simulink model "LUT_liver_pancreas_35"  (R2023b)
settings: Solver=FixedStepAuto  StartTime=0  StopTime=10.1  FixedStep=Timegap  RelTol=1e-3
model workspace (MAT data in the model file):
  T1_input = 1.34
(part 3 of 3)

== system LUT_liver_pancreas_35/If Action Subsystem6/If Action Subsystem2/If Action Subsystem9/If Action Subsystem1 ==
  In1 : Inport
  Action Port : ActionPort  ActionPortLabel=elseif( u1 >= 1.915)
  LUT 1.92RR : Lookup_n-D  NumberOfTableDimensions=1  BreakpointsForDimension1=[404.7876;540.8206;633.9575;726.1135;817.552;908.4902;999.0755;1089.407;1179.553;1269.559;1359.459;1449.276;1539.029;1628.729;1718.387;1808.011;1897.606]  Table=[400;500;600;700;800;900;1000;1100;1200;1300;1400;1500;1600;1700;1800;1900;2000]  InternalRulePriority=Speed  RndMeth=Simplest
  Out1 : Outport
  wires:
  In1/1 -> LUT 1.92RR/1
  LUT 1.92RR/1 -> Out1/1

== system LUT_liver_pancreas_35/If Action Subsystem6/If Action Subsystem2/If Action Subsystem9/If Action Subsystem10 ==
  In1 : Inport
  Action Port : ActionPort  ActionPortLabel=if(u1 >= 1.995)
  LUT 2.00RR : Lookup_n-D  NumberOfTableDimensions=1  BreakpointsForDimension1=[404.3841;540.3186;633.3836;725.4083;816.6655;907.3828;997.7171;1087.775;1177.629;1267.33;1356.913;1446.406;1535.826;1625.189;1714.506;1803.784;1893.031]  Table=[400;500;600;700;800;900;1000;1100;1200;1300;1400;1500;1600;1700;1800;1900;2000]  InternalRulePriority=Speed  RndMeth=Simplest
  Out1 : Outport
  wires:
  In1/1 -> LUT 2.00RR/1
  LUT 2.00RR/1 -> Out1/1

== system LUT_liver_pancreas_35/If Action Subsystem6/If Action Subsystem2/If Action Subsystem9/If Action Subsystem11 ==
  In1 : Inport
  Action Port : ActionPort  ActionPortLabel=elseif( u1 >= 1.905)
  LUT 1.91RR : Lookup_n-D  NumberOfTableDimensions=1  BreakpointsForDimension1=[404.8402;540.8879;634.0358;726.2106;817.6743;908.6425;999.2618;1089.63;1179.815;1269.862;1359.804;1449.664;1539.46;1629.205;1718.908;1808.578;1898.219]  Table=[400;500;600;700;800;900;1000;1100;1200;1300;1400;1500;1600;1700;1800;1900;2000]  InternalRulePriority=Speed  RndMeth=Simplest
  Out1 : Outport
  wires:
  In1/1 -> LUT 1.91RR/1
  LUT 1.91RR/1 -> Out1/1

== system LUT_liver_pancreas_35/If Action Subsystem6/If Action Subsystem2/If Action Subsystem9/If Action Subsystem2 ==
  In1 : Inport
  Action Port : ActionPort  ActionPortLabel=else
  LUT 1.90RR : Lookup_n-D  NumberOfTableDimensions=1  BreakpointsForDimension1=[404.8934;540.9562;634.1157;726.3098;817.7992;908.7982;999.4519;1089.858;1180.082;1270.17;1360.155;1450.058;1539.899;1629.689;1719.438;1809.154;1898.841]  Table=[400;500;600;700;800;900;1000;1100;1200;1300;1400;1500;1600;1700;1800;1900;2000]  InternalRulePriority=Speed  RndMeth=Simplest
  Out1 : Outport
  wires:
  In1/1 -> LUT 1.90RR/1
  LUT 1.90RR/1 -> Out1/1

== system LUT_liver_pancreas_35/If Action Subsystem6/If Action Subsystem2/If Action Subsystem9/If Action Subsystem3 ==
  In1 : Inport
  Action Port : ActionPort  ActionPortLabel=elseif( u1 >= 1.925)
  LUT 1.93RR : Lookup_n-D  NumberOfTableDimensions=1  BreakpointsForDimension1=[404.7354;540.7544;633.8807;726.0185;817.4325;908.341;998.8931;1089.189;1179.296;1269.262;1359.121;1448.895;1538.604;1628.261;1717.874;1807.453;1897.003]  Table=[400;500;600;700;800;900;1000;1100;1200;1300;1400;1500;1600;1700;1800;1900;2000]  InternalRulePriority=Speed  RndMeth=Simplest
  Out1 : Outport
  wires:
  In1/1 -> LUT 1.93RR/1
  LUT 1.93RR/1 -> Out1/1

== system LUT_liver_pancreas_35/If Action Subsystem6/If Action Subsystem2/If Action Subsystem9/If Action Subsystem4 ==
  In1 : Inport
  Action Port : ActionPort  ActionPortLabel=elseif( u1 >= 1.935)
  LUT 1.94RR : Lookup_n-D  NumberOfTableDimensions=1  BreakpointsForDimension1=[404.6838;540.6892;633.8054;725.9255;817.3155;908.1951;998.7144;1088.974;1179.044;1268.97;1358.788;1448.521;1538.187;1627.8;1717.37;1806.904;1896.409]  Table=[400;500;600;700;800;900;1000;1100;1200;1300;1400;1500;1600;1700;1800;1900;2000]  InternalRulePriority=Speed  RndMeth=Simplest
  Out1 : Outport
  wires:
  In1/1 -> LUT 1.94RR/1
  LUT 1.94RR/1 -> Out1/1

== system LUT_liver_pancreas_35/If Action Subsystem6/If Action Subsystem2/If Action Subsystem9/If Action Subsystem5 ==
  In1 : Inport
  Action Port : ActionPort  ActionPortLabel=elseif( u1 >= 1.955)
  LUT 1.96RR : Lookup_n-D  NumberOfTableDimensions=1  BreakpointsForDimension1=[404.582;540.5618;633.6592;725.7455;817.0891;907.9124;998.3679;1088.558;1178.554;1268.403;1358.141;1447.791;1537.374;1626.901;1716.384;1805.831;1895.248]  Table=[400;500;600;700;800;900;1000;1100;1200;1300;1400;1500;1600;1700;1800;1900;2000]  InternalRulePriority=Speed  RndMeth=Simplest
  Out1 : Outport
  wires:
  In1/1 -> LUT 1.96RR/1
  LUT 1.96RR/1 -> Out1/1

== system LUT_liver_pancreas_35/If Action Subsystem6/If Action Subsystem2/If Action Subsystem9/If Action Subsystem6 ==
  In1 : Inport
  Action Port : ActionPort  ActionPortLabel=elseif( u1 >= 1.945)
  LUT 1.95RR : Lookup_n-D  NumberOfTableDimensions=1  BreakpointsForDimension1=[404.6326;540.625;633.7316;725.8345;817.201;908.0522;998.5393;1088.764;1178.796;1268.684;1358.461;1448.153;1537.777;1627.347;1716.873;1806.363;1895.824]  Table=[400;500;600;700;800;900;1000;1100;1200;1300;1400;1500;1600;1700;1800;1900;2000]  InternalRulePriority=Speed  RndMeth=Simplest
  Out1 : Outport
  wires:
  In1/1 -> LUT 1.95RR/1
  LUT 1.95RR/1 -> Out1/1

== system LUT_liver_pancreas_35/If Action Subsystem6/If Action Subsystem2/If Action Subsystem9/If Action Subsystem7 ==
  In1 : Inport
  Action Port : ActionPort  ActionPortLabel=elseif( u1 >= 1.965)
  LUT 1.97RR : Lookup_n-D  NumberOfTableDimensions=1  BreakpointsForDimension1=[404.5318;540.4996;633.5882;725.6584;816.9796;907.7756;998.2001;1088.357;1178.316;1268.127;1357.825;1447.436;1536.977;1626.463;1715.903;1805.307;1894.681]  Table=[400;500;600;700;800;900;1000;1100;1200;1300;1400;1500;1600;1700;1800;1900;2000]  InternalRulePriority=Speed  RndMeth=Simplest
  Out1 : Outport
  wires:
  In1/1 -> LUT 1.97RR/1
  LUT 1.97RR/1 -> Out1/1

== system LUT_liver_pancreas_35/If Action Subsystem6/If Action Subsystem2/If Action Subsystem9/If Action Subsystem8 ==
  In1 : Inport
  Action Port : ActionPort  ActionPortLabel=elseif( u1 >= 1.975)
  LUT 1.98RR : Lookup_n-D  NumberOfTableDimensions=1  BreakpointsForDimension1=[404.4821;540.4383;633.5187;725.5732;816.8726;907.6418;998.0357;1088.159;1178.082;1267.856;1357.516;1447.086;1536.587;1626.031;1715.43;1804.792;1894.123]  Table=[400;500;600;700;800;900;1000;1100;1200;1300;1400;1500;1600;1700;1800;1900;2000]  InternalRulePriority=Speed  RndMeth=Simplest
  Out1 : Outport
  wires:
  In1/1 -> LUT 1.98RR/1
  LUT 1.98RR/1 -> Out1/1

== system LUT_liver_pancreas_35/If Action Subsystem6/If Action Subsystem2/If Action Subsystem9/If Action Subsystem9 ==
  In1 : Inport
  Action Port : ActionPort  ActionPortLabel=elseif(u1 >= 1.985)
  LUT 1.99RR : Lookup_n-D  NumberOfTableDimensions=1  BreakpointsForDimension1=[404.4328;540.378;633.4504;725.4899;816.7679;907.5109;997.8747;1087.965;1177.853;1267.59;1357.212;1446.743;1536.203;1625.607;1714.964;1804.284;1893.573]  Table=[400;500;600;700;800;900;1000;1100;1200;1300;1400;1500;1600;1700;1800;1900;2000]  InternalRulePriority=Speed  RndMeth=Simplest
  Out1 : Outport
  wires:
  In1/1 -> LUT 1.99RR/1
  LUT 1.99RR/1 -> Out1/1

== system LUT_liver_pancreas_35/If Action Subsystem6/If Action Subsystem3/If Action Subsystem5/If Action Subsystem1 ==
  In1 : Inport
  Action Port : ActionPort  ActionPortLabel=elseif( u1 >= 0.615)
  LUT 0.62RR : Lookup_n-D  NumberOfTableDimensions=1  BreakpointsForDimension1=[422.6336;583.5736;694.2332;805.1871;916.263;1027.405;1138.585;1249.783;1360.984;1472.171;1583.31;1694.13;1806.172;1917.097;2028.157;2139.213;2250.242]  Table=[400;500;600;700;800;900;1000;1100;1200;1300;1400;1500;1600;1700;1800;1900;2000]  InternalRulePriority=Speed  RndMeth=Simplest
  Out1 : Outport
  wires:
  In1/1 -> LUT 0.62RR/1
  LUT 0.62RR/1 -> Out1/1

== system LUT_liver_pancreas_35/If Action Subsystem6/If Action Subsystem3/If Action Subsystem5/If Action Subsystem10 ==
  In1 : Inport
  Action Port : ActionPort  ActionPortLabel=elseif( u1 >= 0.605)
  LUT 0.61RR : Lookup_n-D  NumberOfTableDimensions=1  BreakpointsForDimension1=[422.9526;584.7206;695.933;807.4484;919.09;1030.799;1142.546;1254.308;1366.068;1477.806;1589.47;1700.311;1813.447;1924.961;2036.559;2148.143;2259.695]  Table=[400;500;600;700;800;900;1000;1100;1200;1300;1400;1500;1600;1700;1800;1900;2000]  InternalRulePriority=Speed  RndMeth=Simplest
  Out1 : Outport
  wires:
  In1/1 -> LUT 0.61RR/1
  LUT 0.61RR/1 -> Out1/1

== system LUT_liver_pancreas_35/If Action Subsystem6/If Action Subsystem3/If Action Subsystem5/If Action Subsystem2 ==
  In1 : Inport
  Action Port : ActionPort  ActionPortLabel=else
  LUT 0.6RR : Lookup_n-D  NumberOfTableDimensions=1  BreakpointsForDimension1=[423.273;585.8952;697.6778;809.7724;921.9972;1034.291;1146.621;1258.963;1371.298;1483.599;1595.782;1705.399;1820.947;1933.043;2045.189;2157.312;2269.393]  Table=[400;500;600;700;800;900;1000;1100;1200;1300;1400;1500;1600;1700;1800;1900;2000]  InternalRulePriority=Speed  RndMeth=Simplest
  Out1 : Outport
  wires:
  In1/1 -> LUT 0.6RR/1
  LUT 0.6RR/1 -> Out1/1

== system LUT_liver_pancreas_35/If Action Subsystem6/If Action Subsystem3/If Action Subsystem5/If Action Subsystem3 ==
  In1 : Inport
  Action Port : ActionPort  ActionPortLabel=elseif( u1 >= 0.625)
  LUT 0.63RR : Lookup_n-D  NumberOfTableDimensions=1  BreakpointsForDimension1=[422.3166;582.4549;692.5789;802.9886;913.5163;1024.109;1134.74;1245.39;1356.046;1466.695;1577.314;1687.781;1799.151;1909.451;2019.985;2130.523;2241.04]  Table=[400;500;600;700;800;900;1000;1100;1200;1300;1400;1500;1600;1700;1800;1900;2000]  InternalRulePriority=Speed  RndMeth=Simplest
  Out1 : Outport
  wires:
  In1/1 -> LUT 0.63RR/1
  LUT 0.63RR/1 -> Out1/1

== system LUT_liver_pancreas_35/If Action Subsystem6/If Action Subsystem3/If Action Subsystem5/If Action Subsystem4 ==
  In1 : Inport
  Action Port : ActionPort  ActionPortLabel=elseif( u1 >= 0.635)
  LUT 0.64RR : Lookup_n-D  NumberOfTableDimensions=1  BreakpointsForDimension1=[422.0023;581.3647;690.97;800.8527;910.8493;1020.909;1131.007;1241.125;1351.253;1461.377;1571.483;1681.509;1785.582;1902.025;2012.044;2122.075;2232.091]  Table=[400;500;600;700;800;900;1000;1100;1200;1300;1400;1500;1600;1700;1800;1900;2000]  InternalRulePriority=Speed  RndMeth=Simplest
  Out1 : Outport
  wires:
  In1/1 -> LUT 0.64RR/1
  LUT 0.64RR/1 -> Out1/1

== system LUT_liver_pancreas_35/If Action Subsystem6/If Action Subsystem3/If Action Subsystem5/If Action Subsystem5 ==
  In1 : Inport
  Action Port : ActionPort  ActionPortLabel=elseif( u1 >= 0.655)
  LUT 0.66RR : Lookup_n-D  NumberOfTableDimensions=1  BreakpointsForDimension1=[421.3837;579.27;687.8874;796.7656;905.7496;1014.793;1123.873;1232.976;1342.09;1451.208;1560.321;1669.408;1778.206;1887.823;1996.844;2105.898;2214.945]  Table=[400;500;600;700;800;900;1000;1100;1200;1300;1400;1500;1600;1700;1800;1900;2000]  InternalRulePriority=Speed  RndMeth=Simplest
  Out1 : Outport
  wires:
  In1/1 -> LUT 0.66RR/1
  LUT 0.66RR/1 -> Out1/1

== system LUT_liver_pancreas_35/If Action Subsystem6/If Action Subsystem3/If Action Subsystem5/If Action Subsystem6 ==
  In1 : Inport
  Action Port : ActionPort  ActionPortLabel=elseif( u1 >= 0.645)
  LUT 0.65RR : Lookup_n-D  NumberOfTableDimensions=1  BreakpointsForDimension1=[421.6912;580.3031;689.4064;798.7787;908.2609;1017.805;1127.386;1236.988;1346.602;1456.216;1565.819;1675.378;1783.464;1894.816;2004.331;2113.868;2223.393]  Table=[400;500;600;700;800;900;1000;1100;1200;1300;1400;1500;1600;1700;1800;1900;2000]  InternalRulePriority=Speed  RndMeth=Simplest
  Out1 : Outport
  wires:
  In1/1 -> LUT 0.65RR/1
  LUT 0.65RR/1 -> Out1/1

== system LUT_liver_pancreas_35/If Action Subsystem6/If Action Subsystem3/If Action Subsystem5/If Action Subsystem7 ==
  In1 : Inport
  Action Port : ActionPort  ActionPortLabel=elseif( u1 >= 0.665)
  LUT 0.67RR : Lookup_n-D  NumberOfTableDimensions=1  BreakpointsForDimension1=[421.0801;578.2651;686.4124;794.8123;903.3138;1011.873;1120.468;1229.085;1337.715;1446.351;1554.985;1663.605;1772.127;1881.043;1989.578;2098.162;2206.742]  Table=[400;500;600;700;800;900;1000;1100;1200;1300;1400;1500;1600;1700;1800;1900;2000]  InternalRulePriority=Speed  RndMeth=Simplest
  Out1 : Outport
  wires:
  In1/1 -> LUT 0.67RR/1
  LUT 0.67RR/1 -> Out1/1

== system LUT_liver_pancreas_35/If Action Subsystem6/If Action Subsystem3/If Action Subsystem5/If Action Subsystem8 ==
  In1 : Inport
  Action Port : ActionPort  ActionPortLabel=elseif(u1 >= 0.675)
  LUT 0.68RR : Lookup_n-D  NumberOfTableDimensions=1  BreakpointsForDimension1=[420.7806;577.2879;684.9805;792.9173;900.9516;1009.041;1117.166;1225.313;1333.473;1441.641;1549.809;1657.97;1766.09;1874.481;1982.528;2090.655;2198.779]  Table=[400;500;600;700;800;900;1000;1100;1200;1300;1400;1500;1600;1700;1800;1900;2000]  InternalRulePriority=Speed  RndMeth=Simplest
  Out1 : Outport
  wires:
  In1/1 -> LUT 0.68RR/1
  LUT 0.68RR/1 -> Out1/1

== system LUT_liver_pancreas_35/If Action Subsystem6/If Action Subsystem3/If Action Subsystem5/If Action Subsystem9 ==
  In1 : Inport
  Action Port : ActionPort  ActionPortLabel=if(u1 >= 0.685)
  LUT 0.69RR : Lookup_n-D  NumberOfTableDimensions=1  BreakpointsForDimension1=[420.4856;576.3379;683.5906;791.0792;898.661;1006.296;1113.964;1221.655;1329.36;1437.073;1544.789;1652.501;1760.195;1862.439;1975.689;2083.371;2191.052]  Table=[400;500;600;700;800;900;1000;1100;1200;1300;1400;1500;1600;1700;1800;1900;2000]  InternalRulePriority=Speed  RndMeth=Simplest
  Out1 : Outport
  wires:
  In1/1 -> LUT 0.69RR/1
  LUT 0.69RR/1 -> Out1/1

== system LUT_liver_pancreas_35/If Action Subsystem6/If Action Subsystem3/If Action Subsystem6/If Action Subsystem1 ==
  In1 : Inport
  Action Port : ActionPort  ActionPortLabel=elseif( u1 >= 0.515)
  LUT 0.52RR : Lookup_n-D  NumberOfTableDimensions=1  BreakpointsForDimension1=[425.7431;596.0299;712.9409;830.2663;947.7614;1065.323;1182.884;1300.384;1417.721;1534.25;1653.44;1770.224;1887.116;2003.896;2120.516;2236.955;2353.2]  Table=[400;500;600;700;800;900;1000;1100;1200;1300;1400;1500;1600;1700;1800;1900;2000]  InternalRulePriority=Speed  RndMeth=Simplest
  Out1 : Outport
  wires:
  In1/1 -> LUT 0.52RR/1
  LUT 0.52RR/1 -> Out1/1

== system LUT_liver_pancreas_35/If Action Subsystem6/If Action Subsystem3/If Action Subsystem6/If Action Subsystem10 ==
  In1 : Inport
  Action Port : ActionPort  ActionPortLabel=elseif( u1 >= 0.505)
  LUT 0.51RR : Lookup_n-D  NumberOfTableDimensions=1  BreakpointsForDimension1=[426.0152;597.3196;714.917;832.9499;951.1599;1069.435;1187.698;1305.881;1423.854;1540.583;1660.719;1778.215;1895.688;2013.001;2130.113;2247.006;2363.667]  Table=[400;500;600;700;800;900;1000;1100;1200;1300;1400;1500;1600;1700;1800;1900;2000]  InternalRulePriority=Speed  RndMeth=Simplest
  Out1 : Outport
  wires:
  In1/1 -> LUT 0.51RR/1
  LUT 0.51RR/1 -> Out1/1

== system LUT_liver_pancreas_35/If Action Subsystem6/If Action Subsystem3/If Action Subsystem6/If Action Subsystem2 ==
  In1 : Inport
  Action Port : ActionPort  ActionPortLabel=else
  LUT 0.50RR : Lookup_n-D  NumberOfTableDimensions=1  BreakpointsForDimension1=[426.2724;598.586;716.8671;835.6082;954.5351;1073.524;1192.49;1311.353;1429.951;1547.041;1667.958;1786.098;1904.115;2021.919;2139.477;2256.768;2373.782]  Table=[400;500;600;700;800;900;1000;1100;1200;1300;1400;1500;1600;1700;1800;1900;2000]  InternalRulePriority=Speed  RndMeth=Simplest
  Out1 : Outport
  wires:
  In1/1 -> LUT 0.50RR/1
  LUT 0.50RR/1 -> Out1/1

== system LUT_liver_pancreas_35/If Action Subsystem6/If Action Subsystem3/If Action Subsystem6/If Action Subsystem3 ==
  In1 : Inport
  Action Port : ActionPort  ActionPortLabel=elseif( u1 >= 0.525)
  LUT 0.53RR : Lookup_n-D  NumberOfTableDimensions=1  BreakpointsForDimension1=[424.9443;594.7286;710.9561;827.5799;944.3669;1061.222;1178.086;1294.904;1411.598;1527.786;1646.232;1762.207;1878.492;1994.71;2110.804;2226.749;2342.533]  Table=[400;500;600;700;800;900;1000;1100;1200;1300;1400;1500;1600;1700;1800;1900;2000]  InternalRulePriority=Speed  RndMeth=Simplest
  Out1 : Outport
  wires:
  In1/1 -> LUT 0.53RR/1
  LUT 0.53RR/1 -> Out1/1

== system LUT_liver_pancreas_35/If Action Subsystem6/If Action Subsystem3/If Action Subsystem6/If Action Subsystem4 ==
  In1 : Inport
  Action Port : ActionPort  ActionPortLabel=elseif( u1 >= 0.535)
  LUT 0.54RR : Lookup_n-D  NumberOfTableDimensions=1  BreakpointsForDimension1=[425.2839;593.4253;708.9767;824.9086;940.9979;1057.157;1173.331;1289.473;1405.522;1521.245;1639.267;1754.228;1869.886;1985.525;2101.069;2216.493;2331.782]  Table=[400;500;600;700;800;900;1000;1100;1200;1300;1400;1500;1600;1700;1800;1900;2000]  InternalRulePriority=Speed  RndMeth=Simplest
  Out1 : Outport
  wires:
  In1/1 -> LUT 0.54RR/1
  LUT 0.54RR/1 -> Out1/1

== system LUT_liver_pancreas_35/If Action Subsystem6/If Action Subsystem3/If Action Subsystem6/If Action Subsystem5 ==
  In1 : Inport
  Action Port : ActionPort  ActionPortLabel=elseif( u1 >= 0.555)
  LUT 0.56RR : Lookup_n-D  NumberOfTableDimensions=1  BreakpointsForDimension1=[424.5481;590.8416;705.0753;819.6628;934.3976;1049.203;1164.034;1278.855;1393.626;1508.247;1621.489;1738.584;1852.937;1967.393;2081.803;2196.135;2310.376]  Table=[400;500;600;700;800;900;1000;1100;1200;1300;1400;1500;1600;1700;1800;1900;2000]  InternalRulePriority=Speed  RndMeth=Simplest
  Out1 : Outport
  wires:
  In1/1 -> LUT 0.56RR/1
  LUT 0.56RR/1 -> Out1/1

== system LUT_liver_pancreas_35/If Action Subsystem6/If Action Subsystem3/If Action Subsystem6/If Action Subsystem6 ==
  In1 : Inport
  Action Port : ActionPort  ActionPortLabel=elseif( u1 >= 0.545)
  LUT 0.55RR : Lookup_n-D  NumberOfTableDimensions=1  BreakpointsForDimension1=[424.8587;592.1276;707.0136;822.2661;937.6706;1053.146;1168.641;1284.117;1399.524;1514.713;1627.08;1746.339;1861.354;1976.403;2091.384;2206.268;2321.04]  Table=[400;500;600;700;800;900;1000;1100;1200;1300;1400;1500;1600;1700;1800;1900;2000]  InternalRulePriority=Speed  RndMeth=Simplest
  Out1 : Outport
  wires:
  In1/1 -> LUT 0.55RR/1
  LUT 0.55RR/1 -> Out1/1

== system LUT_liver_pancreas_35/If Action Subsystem6/If Action Subsystem3/If Action Subsystem6/If Action Subsystem7 ==
  In1 : Inport
  Action Port : ActionPort  ActionPortLabel=elseif( u1 >= 0.565)
  LUT 0.57RR : Lookup_n-D  NumberOfTableDimensions=1  BreakpointsForDimension1=[424.2327;589.5721;703.1683;817.1068;931.1881;1045.34;1159.521;1273.7;1387.844;1501.884;1615.274;1731.006;1844.668;1958.528;2072.366;2186.143;2299.845]  Table=[400;500;600;700;800;900;1000;1100;1200;1300;1400;1500;1600;1700;1800;1900;2000]  InternalRulePriority=Speed  RndMeth=Simplest
  Out1 : Outport
  wires:
  In1/1 -> LUT 0.57RR/1
  LUT 0.57RR/1 -> Out1/1

== system LUT_liver_pancreas_35/If Action Subsystem6/If Action Subsystem3/If Action Subsystem6/If Action Subsystem8 ==
  In1 : Inport
  Action Port : ActionPort  ActionPortLabel=elseif(u1 >= 0.575)
  LUT 0.58RR : Lookup_n-D  NumberOfTableDimensions=1  BreakpointsForDimension1=[423.9142;588.3227;701.2975;814.6039;928.0487;1041.564;1155.111;1268.662;1382.19;1495.645;1608.761;1723.669;1836.569;1949.837;2063.105;2176.326;2289.486]  Table=[400;500;600;700;800;900;1000;1100;1200;1300;1400;1500;1600;1700;1800;1900;2000]  InternalRulePriority=Speed  RndMeth=Simplest
  Out1 : Outport
  wires:
  In1/1 -> LUT 0.58RR/1
  LUT 0.58RR/1 -> Out1/1

== system LUT_liver_pancreas_35/If Action Subsystem6/If Action Subsystem3/If Action Subsystem6/If Action Subsystem9 ==
  In1 : Inport
  Action Port : ActionPort  ActionPortLabel=if(u1 >= 0.585)
  LUT 0.59RR : Lookup_n-D  NumberOfTableDimensions=1  BreakpointsForDimension1=[423.5939;587.0964;699.4665;812.1582;924.9841;1037.88;1150.81;1263.749;1376.673;1489.547;1602.227;1709.092;1828.658;1941.338;2054.041;2166.71;2279.328]  Table=[400;500;600;700;800;900;1000;1100;1200;1300;1400;1500;1600;1700;1800;1900;2000]  InternalRulePriority=Speed  RndMeth=Simplest
  Out1 : Outport
  wires:
  In1/1 -> LUT 0.59RR/1
  LUT 0.59RR/1 -> Out1/1

== system LUT_liver_pancreas_35/If Action Subsystem6/If Action Subsystem3/If Action Subsystem7/If Action Subsystem1 ==
  In1 : Inport
  Action Port : ActionPort  ActionPortLabel=elseif( u1 >= 0.715)
  LUT 0.72RR : Lookup_n-D  NumberOfTableDimensions=1  BreakpointsForDimension1=[419.6278;573.6455;679.6626;785.8906;892.1983;998.5516;1104.935;1211.338;1317.756;1424.183;1530.616;1637.051;1743.486;1849.909;1956.375;2062.793;2169.214]  Table=[400;500;600;700;800;900;1000;1100;1200;1300;1400;1500;1600;1700;1800;1900;2000]  InternalRulePriority=Speed  RndMeth=Simplest
  Out1 : Outport
  wires:
  In1/1 -> LUT 0.72RR/1
  LUT 0.72RR/1 -> Out1/1

== system LUT_liver_pancreas_35/If Action Subsystem6/If Action Subsystem3/If Action Subsystem7/If Action Subsystem10 ==
  In1 : Inport
  Action Port : ActionPort  ActionPortLabel=elseif( u1 >= 0.705)
  LUT 0.71RR : Lookup_n-D  NumberOfTableDimensions=1  BreakpointsForDimension1=[419.909;574.5174;680.9328;787.5675;894.2865;1001.054;1107.852;1214.672;1321.506;1428.349;1535.197;1642.046;1748.892;1855.694;1962.619;2069.446;2176.275]  Table=[400;500;600;700;800;900;1000;1100;1200;1300;1400;1500;1600;1700;1800;1900;2000]  InternalRulePriority=Speed  RndMeth=Simplest
  Out1 : Outport
  wires:
  In1/1 -> LUT 0.71RR/1
  LUT 0.71RR/1 -> Out1/1

== system LUT_liver_pancreas_35/If Action Subsystem6/If Action Subsystem3/If Action Subsystem7/If Action Subsystem2 ==
  In1 : Inport
  Action Port : ActionPort  ActionPortLabel=else
  LUT 0.70RR : Lookup_n-D  NumberOfTableDimensions=1  BreakpointsForDimension1=[420.195;575.4146;682.2417;789.2965;896.4401;1003.634;1110.861;1218.109;1325.372;1432.644;1539.919;1647.194;1754.461;1861.375;1969.055;2076.303;2183.552]  Table=[400;500;600;700;800;900;1000;1100;1200;1300;1400;1500;1600;1700;1800;1900;2000]  InternalRulePriority=Speed  RndMeth=Simplest
  Out1 : Outport
  wires:
  In1/1 -> LUT 0.70RR/1
  LUT 0.70RR/1 -> Out1/1

== system LUT_liver_pancreas_35/If Action Subsystem6/If Action Subsystem3/If Action Subsystem7/If Action Subsystem3 ==
  In1 : Inport
  Action Port : ActionPort  ActionPortLabel=elseif( u1 >= 0.725)
  LUT 0.73RR : Lookup_n-D  NumberOfTableDimensions=1  BreakpointsForDimension1=[419.3512;572.7984;678.4301;784.2641;890.1733;996.1255;1102.106;1208.106;1314.12;1420.143;1526.173;1632.205;1738.239;1844.269;1950.317;2056.338;2162.36]  Table=[400;500;600;700;800;900;1000;1100;1200;1300;1400;1500;1600;1700;1800;1900;2000]  InternalRulePriority=Speed  RndMeth=Simplest
  Out1 : Outport
  wires:
  In1/1 -> LUT 0.73RR/1
  LUT 0.73RR/1 -> Out1/1

== system LUT_liver_pancreas_35/If Action Subsystem6/If Action Subsystem3/If Action Subsystem7/If Action Subsystem4 ==
  In1 : Inport
  Action Port : ActionPort  ActionPortLabel=elseif( u1 >= 0.735)
  LUT 0.74RR : Lookup_n-D  NumberOfTableDimensions=1  BreakpointsForDimension1=[419.0794;571.9752;677.234;782.6864;888.2094;993.7726;1099.362;1204.971;1310.593;1416.224;1521.862;1627.503;1733.147;1838.789;1939.661;2050.073;2155.709]  Table=[400;500;600;700;800;900;1000;1100;1200;1300;1400;1500;1600;1700;1800;1900;2000]  InternalRulePriority=Speed  RndMeth=Simplest
  Out1 : Outport
  wires:
  In1/1 -> LUT 0.74RR/1
  LUT 0.74RR/1 -> Out1/1

== system LUT_liver_pancreas_35/If Action Subsystem6/If Action Subsystem3/If Action Subsystem7/If Action Subsystem5 ==
  In1 : Inport
  Action Port : ActionPort  ActionPortLabel=elseif( u1 >= 0.755)
  LUT 0.76RR : Lookup_n-D  NumberOfTableDimensions=1  BreakpointsForDimension1=[418.5498;570.398;674.9465;779.6711;884.4567;989.2767;1094.12;1198.98;1303.852;1408.734;1513.621;1618.513;1723.407;1828.302;1933.195;2038.092;2142.984]  Table=[400;500;600;700;800;900;1000;1100;1200;1300;1400;1500;1600;1700;1800;1900;2000]  InternalRulePriority=Speed  RndMeth=Simplest
  Out1 : Outport
  wires:
  In1/1 -> LUT 0.76RR/1
  LUT 0.76RR/1 -> Out1/1

== system LUT_liver_pancreas_35/If Action Subsystem6/If Action Subsystem3/If Action Subsystem7/If Action Subsystem6 ==
  In1 : Inport
  Action Port : ActionPort  ActionPortLabel=elseif( u1 >= 0.745)
  LUT 0.75RR : Lookup_n-D  NumberOfTableDimensions=1  BreakpointsForDimension1=[418.8123;571.1753;676.0732;781.156;886.3045;991.4905;1096.701;1201.93;1307.172;1412.423;1517.68;1622.941;1728.204;1833.468;1938.732;2043.993;2149.252]  Table=[400;500;600;700;800;900;1000;1100;1200;1300;1400;1500;1600;1700;1800;1900;2000]  InternalRulePriority=Speed  RndMeth=Simplest
  Out1 : Outport
  wires:
  In1/1 -> LUT 0.75RR/1
  LUT 0.75RR/1 -> Out1/1

== system LUT_liver_pancreas_35/If Action Subsystem6/If Action Subsystem3/If Action Subsystem7/If Action Subsystem7 ==
  In1 : Inport
  Action Port : ActionPort  ActionPortLabel=elseif( u1 >= 0.765)
  LUT 0.77RR : Lookup_n-D  NumberOfTableDimensions=1  BreakpointsForDimension1=[418.2921;569.6426;673.8529;778.2303;882.6638;987.1289;1091.615;1196.117;1300.631;1405.153;1509.682;1614.214;1718.749;1823.285;1927.819;2032.366;2136.897]  Table=[400;500;600;700;800;900;1000;1100;1200;1300;1400;1500;1600;1700;1800;1900;2000]  InternalRulePriority=Speed  RndMeth=Simplest
  Out1 : Outport
  wires:
  In1/1 -> LUT 0.77RR/1
  LUT 0.77RR/1 -> Out1/1

== system LUT_liver_pancreas_35/If Action Subsystem6/If Action Subsystem3/If Action Subsystem7/If Action Subsystem8 ==
  In1 : Inport
  Action Port : ActionPort  ActionPortLabel=elseif(u1 >= 0.775)
  LUT 0.78RR : Lookup_n-D  NumberOfTableDimensions=1  BreakpointsForDimension1=[418.0389;568.9084;672.7912;776.8321;880.9241;985.0446;1089.185;1193.339;1297.504;1401.678;1505.857;1610.041;1714.227;1818.414;1922.598;2026.814;2130.987]  Table=[400;500;600;700;800;900;1000;1100;1200;1300;1400;1500;1600;1700;1800;1900;2000]  InternalRulePriority=Speed  RndMeth=Simplest
  Out1 : Outport
  wires:
  In1/1 -> LUT 0.78RR/1
  LUT 0.78RR/1 -> Out1/1

== system LUT_liver_pancreas_35/If Action Subsystem6/If Action Subsystem3/If Action Subsystem7/If Action Subsystem9 ==
  In1 : Inport
  Action Port : ActionPort  ActionPortLabel=if(u1 >= 0.785)
  LUT 0.79RR : Lookup_n-D  NumberOfTableDimensions=1  BreakpointsForDimension1=[417.7903;568.1947;671.7604;775.475;879.2356;983.0216;1086.825;1190.642;1294.469;1398.303;1502.144;1605.988;1709.835;1813.682;1917.527;2017.191;2125.247]  Table=[400;500;600;700;800;900;1000;1100;1200;1300;1400;1500;1600;1700;1800;1900;2000]  InternalRulePriority=Speed  RndMeth=Simplest
  Out1 : Outport
  wires:
  In1/1 -> LUT 0.79RR/1
  LUT 0.79RR/1 -> Out1/1

== system LUT_liver_pancreas_35/If Action Subsystem6/If Action Subsystem3/If Action Subsystem8/If Action Subsystem1 ==
  In1 : Inport
  Action Port : ActionPort  ActionPortLabel=elseif( u1 >= 0.815)
  LUT 0.82RR : Lookup_n-D  NumberOfTableDimensions=1  BreakpointsForDimension1=[417.0711;566.1704;668.8427;771.6361;874.4597;977.2991;1080.15;1183.01;1285.877;1388.751;1491.629;1594.51;1697.393;1800.278;1903.159;2006.015;2109.009]  Table=[400;500;600;700;800;900;1000;1100;1200;1300;1400;1500;1600;1700;1800;1900;2000]  InternalRulePriority=Speed  RndMeth=Simplest
  Out1 : Outport
  wires:
  In1/1 -> LUT 0.82RR/1
  LUT 0.82RR/1 -> Out1/1

== system LUT_liver_pancreas_35/If Action Subsystem6/If Action Subsystem3/If Action Subsystem8/If Action Subsystem10 ==
  In1 : Inport
  Action Port : ActionPort  ActionPortLabel=elseif( u1 >= 0.805)
  LUT 0.81RR : Lookup_n-D  NumberOfTableDimensions=1  BreakpointsForDimension1=[417.3065;566.8263;669.7871;772.8783;876.0051;979.1509;1082.31;1185.48;1288.659;1391.843;1495.033;1598.227;1701.422;1804.619;1907.813;2010.965;2114.259]  Table=[400;500;600;700;800;900;1000;1100;1200;1300;1400;1500;1600;1700;1800;1900;2000]  InternalRulePriority=Speed  RndMeth=Simplest
  Out1 : Outport
  wires:
  In1/1 -> LUT 0.81RR/1
  LUT 0.81RR/1 -> Out1/1

== system LUT_liver_pancreas_35/If Action Subsystem6/If Action Subsystem3/If Action Subsystem8/If Action Subsystem2 ==
  In1 : Inport
  Action Port : ActionPort  ActionPortLabel=else
  LUT 0.80RR : Lookup_n-D  NumberOfTableDimensions=1  BreakpointsForDimension1=[417.5462;567.5009;670.7593;774.1575;877.5965;981.0577;1084.535;1188.023;1291.521;1395.026;1498.537;1602.051;1705.568;1809.086;1912.6;2016.004;2119.672]  Table=[400;500;600;700;800;900;1000;1100;1200;1300;1400;1500;1600;1700;1800;1900;2000]  InternalRulePriority=Speed  RndMeth=Simplest
  Out1 : Outport
  wires:
  In1/1 -> LUT 0.80RR/1
  LUT 0.80RR/1 -> Out1/1

== system LUT_liver_pancreas_35/If Action Subsystem6/If Action Subsystem3/If Action Subsystem8/If Action Subsystem3 ==
  In1 : Inport
  Action Port : ActionPort  ActionPortLabel=elseif( u1 >= 0.825)
  LUT 0.83RR : Lookup_n-D  NumberOfTableDimensions=1  BreakpointsForDimension1=[416.84;565.5324;667.9252;770.4296;872.9586;975.5002;1078.051;1180.61;1283.175;1385.745;1488.32;1590.897;1693.477;1796.057;1898.635;2001.195;2103.941]  Table=[400;500;600;700;800;900;1000;1100;1200;1300;1400;1500;1600;1700;1800;1900;2000]  InternalRulePriority=Speed  RndMeth=Simplest
  Out1 : Outport
  wires:
  In1/1 -> LUT 0.83RR/1
  LUT 0.83RR/1 -> Out1/1

== system LUT_liver_pancreas_35/If Action Subsystem6/If Action Subsystem3/If Action Subsystem8/If Action Subsystem4 ==
  In1 : Inport
  Action Port : ActionPort  ActionPortLabel=elseif( u1 >= 0.835)
  LUT 0.84RR : Lookup_n-D  NumberOfTableDimensions=1  BreakpointsForDimension1=[416.6131;564.9118;667.0337;769.2574;871.5004;973.7526;1076.012;1178.277;1280.548;1382.824;1485.103;1587.385;1689.669;1791.953;1894.236;1996.504;2095.038]  Table=[400;500;600;700;800;900;1000;1100;1200;1300;1400;1500;1600;1700;1800;1900;2000]  InternalRulePriority=Speed  RndMeth=Simplest
  Out1 : Outport
  wires:
  In1/1 -> LUT 0.84RR/1
  LUT 0.84RR/1 -> Out1/1

== system LUT_liver_pancreas_35/If Action Subsystem6/If Action Subsystem3/If Action Subsystem8/If Action Subsystem5 ==
  In1 : Inport
  Action Port : ActionPort  ActionPortLabel=elseif( u1 >= 0.855)
  LUT 0.86RR : Lookup_n-D  NumberOfTableDimensions=1  BreakpointsForDimension1=[416.1714;563.7206;665.325;767.0117;868.7065;970.4035;1072.103;1173.806;1275.512;1377.222;1478.933;1580.648;1682.363;1784.079;1885.793;1987.497;2089.104]  Table=[400;500;600;700;800;900;1000;1100;1200;1300;1400;1500;1600;1700;1800;1900;2000]  InternalRulePriority=Speed  RndMeth=Simplest
  Out1 : Outport
  wires:
  In1/1 -> LUT 0.86RR/1
  LUT 0.86RR/1 -> Out1/1

== system LUT_liver_pancreas_35/If Action Subsystem6/If Action Subsystem3/If Action Subsystem8/If Action Subsystem6 ==
  In1 : Inport
  Action Port : ActionPort  ActionPortLabel=elseif( u1 >= 0.845)
  LUT 0.85RR : Lookup_n-D  NumberOfTableDimensions=1  BreakpointsForDimension1=[416.3902;564.308;666.1672;768.1185;870.0835;972.0542;1074.03;1176.01;1277.995;1379.984;1481.975;1583.97;1685.966;1787.962;1889.956;1991.939;2093.654]  Table=[400;500;600;700;800;900;1000;1100;1200;1300;1400;1500;1600;1700;1800;1900;2000]  InternalRulePriority=Speed  RndMeth=Simplest
  Out1 : Outport
  wires:
  In1/1 -> LUT 0.85RR/1
  LUT 0.85RR/1 -> Out1/1

== system LUT_liver_pancreas_35/If Action Subsystem6/If Action Subsystem3/If Action Subsystem8/If Action Subsystem7 ==
  In1 : Inport
  Action Port : ActionPort  ActionPortLabel=elseif( u1 >= 0.865)
  LUT 0.87RR : Lookup_n-D  NumberOfTableDimensions=1  BreakpointsForDimension1=[415.9566;563.1488;664.5062;765.9359;867.368;968.7987;1070.23;1171.662;1273.097;1374.535;1475.974;1577.415;1678.857;1780.3;1881.741;1983.174;2084.552]  Table=[400;500;600;700;800;900;1000;1100;1200;1300;1400;1500;1600;1700;1800;1900;2000]  InternalRulePriority=Speed  RndMeth=Simplest
  Out1 : Outport
  wires:
  In1/1 -> LUT 0.87RR/1
  LUT 0.87RR/1 -> Out1/1

== system LUT_liver_pancreas_35/If Action Subsystem6/If Action Subsystem3/If Action Subsystem8/If Action Subsystem8 ==
  In1 : Inport
  Action Port : ActionPort  ActionPortLabel=elseif(u1 >= 0.875)
  LUT 0.88RR : Lookup_n-D  NumberOfTableDimensions=1  BreakpointsForDimension1=[415.7455;562.5923;663.71;764.89;866.0666;967.2382;1068.408;1169.578;1270.748;1371.921;1473.095;1574.27;1675.446;1776.622;1877.796;1978.964;2080.096]  Table=[400;500;600;700;800;900;1000;1100;1200;1300;1400;1500;1600;1700;1800;1900;2000]  InternalRulePriority=Speed  RndMeth=Simplest
  Out1 : Outport
  wires:
  In1/1 -> LUT 0.88RR/1
  LUT 0.88RR/1 -> Out1/1

== system LUT_liver_pancreas_35/If Action Subsystem6/If Action Subsystem3/If Action Subsystem8/If Action Subsystem9 ==
  In1 : Inport
  Action Port : ActionPort  ActionPortLabel=if(u1 >= 0.885)
  LUT 0.89RR : Lookup_n-D  NumberOfTableDimensions=1  BreakpointsForDimension1=[415.5383;562.0505;662.9356;763.873;864.8011;965.7205;1066.636;1167.549;1268.463;1369.377;1470.292;1571.208;1672.125;1773.041;1873.956;1974.865;2075.748]  Table=[400;500;600;700;800;900;1000;1100;1200;1300;1400;1500;1600;1700;1800;1900;2000]  InternalRulePriority=Speed  RndMeth=Simplest
  Out1 : Outport
  wires:
  In1/1 -> LUT 0.89RR/1
  LUT 0.89RR/1 -> Out1/1

== system LUT_liver_pancreas_35/If Action Subsystem6/If Action Subsystem3/If Action Subsystem9/If Action Subsystem1 ==
  In1 : Inport
  Action Port : ActionPort  ActionPortLabel=elseif( u1 >= 0.915)
  LUT 0.92RR : Lookup_n-D  NumberOfTableDimensions=1  BreakpointsForDimension1=[414.9383;560.5088;660.7364;760.9857;861.2077;961.4098;1061.6;1161.784;1261.964;1362.142;1462.319;1562.496;1662.672;1762.848;1863.022;1963.192;2063.35]  Table=[400;500;600;700;800;900;1000;1100;1200;1300;1400;1500;1600;1700;1800;1900;2000]  InternalRulePriority=Speed  RndMeth=Simplest
  Out1 : Outport
  wires:
  In1/1 -> LUT 0.92RR/1
  LUT 0.92RR/1 -> Out1/1

== system LUT_liver_pancreas_35/If Action Subsystem6/If Action Subsystem3/If Action Subsystem9/If Action Subsystem10 ==
  In1 : Inport
  Action Port : ActionPort  ActionPortLabel=elseif( u1 >= 0.905)
  LUT 0.91RR : Lookup_n-D  NumberOfTableDimensions=1  BreakpointsForDimension1=[415.1347;561.0092;661.4495;761.9217;862.3728;962.8077;1063.233;1163.654;1264.072;1364.49;1464.907;1565.324;1665.741;1766.157;1866.572;1966.983;2067.378]  Table=[400;500;600;700;800;900;1000;1100;1200;1300;1400;1500;1600;1700;1800;1900;2000]  InternalRulePriority=Speed  RndMeth=Simplest
  Out1 : Outport
  wires:
  In1/1 -> LUT 0.91RR/1
  LUT 0.91RR/1 -> Out1/1

== system LUT_liver_pancreas_35/If Action Subsystem6/If Action Subsystem3/If Action Subsystem9/If Action Subsystem2 ==
  In1 : Inport
  Action Port : ActionPort  ActionPortLabel=else
  LUT 0.90RR : Lookup_n-D  NumberOfTableDimensions=1  BreakpointsForDimension1=[415.3347;561.523;662.1823;762.8839;863.5702;964.2442;1064.911;1165.575;1266.238;1366.901;1467.563;1568.227;1668.891;1769.554;1870.216;1970.872;2071.51]  Table=[400;500;600;700;800;900;1000;1100;1200;1300;1400;1500;1600;1700;1800;1900;2000]  InternalRulePriority=Speed  RndMeth=Simplest
  Out1 : Outport
  wires:
  In1/1 -> LUT 0.90RR/1
  LUT 0.90RR/1 -> Out1/1

== system LUT_liver_pancreas_35/If Action Subsystem6/If Action Subsystem3/If Action Subsystem9/If Action Subsystem3 ==
  In1 : Inport
  Action Port : ActionPort  ActionPortLabel=elseif( u1 >= 0.925)
  LUT 0.93RR : Lookup_n-D  NumberOfTableDimensions=1  BreakpointsForDimension1=[414.7452;560.0213;660.0424;760.0748;860.0738;960.0491;1060.01;1159.963;1259.91;1359.855;1459.798;1559.741;1659.683;1759.623;1859.562;1959.498;2059.423]  Table=[400;500;600;700;800;900;1000;1100;1200;1300;1400;1500;1600;1700;1800;1900;2000]  InternalRulePriority=Speed  RndMeth=Simplest
  Out1 : Outport
  wires:
  In1/1 -> LUT 0.93RR/1
  LUT 0.93RR/1 -> Out1/1

== system LUT_liver_pancreas_35/If Action Subsystem6/If Action Subsystem3/If Action Subsystem9/If Action Subsystem4 ==
  In1 : Inport
  Action Port : ActionPort  ActionPortLabel=elseif( u1 >= 0.935)
  LUT 0.94RR : Lookup_n-D  NumberOfTableDimensions=1  BreakpointsForDimension1=[414.5556;559.5463;659.3669;759.1883;858.9701;958.7244;1058.462;1158.189;1257.91;1357.627;1457.342;1557.056;1656.769;1756.48;1856.19;1955.896;2055.593]  Table=[400;500;600;700;800;900;1000;1100;1200;1300;1400;1500;1600;1700;1800;1900;2000]  InternalRulePriority=Speed  RndMeth=Simplest
  Out1 : Outport
  wires:
  In1/1 -> LUT 0.94RR/1
  LUT 0.94RR/1 -> Out1/1

== system LUT_liver_pancreas_35/If Action Subsystem6/If Action Subsystem3/If Action Subsystem9/If Action Subsystem5 ==
  In1 : Inport
  Action Port : ActionPort  ActionPortLabel=elseif( u1 >= 0.955)
  LUT 0.96RR : Lookup_n-D  NumberOfTableDimensions=1  BreakpointsForDimension1=[414.1861;558.6322;658.0688;757.4851;856.8494;956.1782;1055.485;1154.778;1254.062;1353.34;1452.615;1551.888;1651.158;1750.427;1849.694;1948.958;2048.215]  Table=[400;500;600;700;800;900;1000;1100;1200;1300;1400;1500;1600;1700;1800;1900;2000]  InternalRulePriority=Speed  RndMeth=Simplest
  Out1 : Outport
  wires:
  In1/1 -> LUT 0.96RR/1
  LUT 0.96RR/1 -> Out1/1

== system LUT_liver_pancreas_35/If Action Subsystem6/If Action Subsystem3/If Action Subsystem9/If Action Subsystem6 ==
  In1 : Inport
  Action Port : ActionPort  ActionPortLabel=elseif( u1 >= 0.945)
  LUT 0.95RR : Lookup_n-D  NumberOfTableDimensions=1  BreakpointsForDimension1=[414.3693;559.0834;658.7092;758.3253;857.8957;957.4345;1056.954;1156.461;1255.961;1355.456;1454.949;1554.439;1653.928;1753.416;1852.901;1952.384;2051.859]  Table=[400;500;600;700;800;900;1000;1100;1200;1300;1400;1500;1600;1700;1800;1900;2000]  InternalRulePriority=Speed  RndMeth=Simplest
  Out1 : Outport
  wires:
  In1/1 -> LUT 0.95RR/1
  LUT 0.95RR/1 -> Out1/1

== system LUT_liver_pancreas_35/If Action Subsystem6/If Action Subsystem3/If Action Subsystem9/If Action Subsystem7 ==
  In1 : Inport
  Action Port : ActionPort  ActionPortLabel=elseif( u1 >= 0.965)
  LUT 0.97RR : Lookup_n-D  NumberOfTableDimensions=1  BreakpointsForDimension1=[414.0061;558.1923;657.4451;756.667;855.8305;954.9545;1054.054;1153.137;1252.21;1351.277;1450.34;1549.4;1648.457;1747.513;1846.566;1945.616;2044.66]  Table=[400;500;600;700;800;900;1000;1100;1200;1300;1400;1500;1600;1700;1800;1900;2000]  InternalRulePriority=Speed  RndMeth=Simplest
  Out1 : Outport
  wires:
  In1/1 -> LUT 0.97RR/1
  LUT 0.97RR/1 -> Out1/1

== system LUT_liver_pancreas_35/If Action Subsystem6/If Action Subsystem3/If Action Subsystem9/If Action Subsystem8 ==
  In1 : Inport
  Action Port : ActionPort  ActionPortLabel=elseif(u1 >= 0.975)
  LUT 0.98RR : Lookup_n-D  NumberOfTableDimensions=1  BreakpointsForDimension1=[413.8292;557.7634;656.8375;755.8701;854.838;953.7622;1052.659;1151.538;1250.406;1349.266;1448.121;1546.973;1645.822;1744.669;1843.514;1942.355;2041.191]  Table=[400;500;600;700;800;900;1000;1100;1200;1300;1400;1500;1600;1700;1800;1900;2000]  InternalRulePriority=Speed  RndMeth=Simplest
  Out1 : Outport
  wires:
  In1/1 -> LUT 0.98RR/1
  LUT 0.98RR/1 -> Out1/1

== system LUT_liver_pancreas_35/If Action Subsystem6/If Action Subsystem3/If Action Subsystem9/If Action Subsystem9 ==
  In1 : Inport
  Action Port : ActionPort  ActionPortLabel=if(u1 >= 0.985)
  LUT 0.99RR : Lookup_n-D  NumberOfTableDimensions=1  BreakpointsForDimension1=[413.6553;557.3452;656.2457;755.094;853.8711;952.6004;1051.299;1149.979;1248.646;1347.304;1445.957;1544.606;1643.251;1741.894;1840.535;1939.172;2037.805]  Table=[400;500;600;700;800;900;1000;1100;1200;1300;1400;1500;1600;1700;1800;1900;2000]  InternalRulePriority=Speed  RndMeth=Simplest
  Out1 : Outport
  wires:
  In1/1 -> LUT 0.99RR/1
  LUT 0.99RR/1 -> Out1/1
